simulink model "Model_Maxime"  (R2023b)
settings: Solver=VariableStepAuto  StartTime=0.0  StopTime=T_tot  FixedStep=1e-6  MaxStep=1/50/100  RelTol=1e-3
values from neighbouring files (symbols this model uses):
  B = 0.0129    [PARAMETERS_MODEL_GR2.m]    (also in Parameters.m; Parameters_Chloe.m)
  d_duration_down_slope = 1    [Parameters.m]    (also in Parameters_Chloe.m)
  d_duration_upslope = 1    [Parameters.m]    (also in Parameters_Chloe.m)
  d_start = 0.5    [Parameters.m]    (also in Parameters_Chloe.m)
  d_start_down_slope = 8    [Parameters.m]    (also in Parameters_Chloe.m)
  d_start_down_step = 11    [Parameters.m]    (also in Parameters_Chloe.m)
  d_start_upslope = 1    [Parameters.m]    (also in Parameters_Chloe.m)
  d_start_upstep = 4    [Parameters.m]    (also in Parameters_Chloe.m)
  d_stop = 2    [Parameters.m]    (also in Parameters_Chloe.m)
  f_r = 50    [PARAMETERS_MODEL_GR2.m]    (also in Parameters.m; Parameters_Chloe.m)
  J = 0.2799    [PARAMETERS_MODEL_GR2.m]    (also in Parameters.m; Parameters_Chloe.m)
  Ki = Ki*Ts_w    (= 0.00645)    [PARAMETERS_MODEL_GR2.m]    (also in Parameters.m = 0.37903125; Parameters_Chloe.m = 1.04185)
  Kp = Kp + Ki*Ts_w/2    (= 210.627975)    [PARAMETERS_MODEL_GR2.m]    (also in Parameters.m = 2.463703125; Parameters_Chloe.m = 6.772025)
  L_lr = 1.8e-3    (= 0.0018)    [PARAMETERS_MODEL_GR2.m]    (also in Parameters.m; Parameters_Chloe.m)
  L_ls = 1.8e-3    (= 0.0018)    [PARAMETERS_MODEL_GR2.m]    (also in Parameters.m; Parameters_Chloe.m)
  N_steady = N_r    (= 1460)    [PARAMETERS_MODEL_GR2.m]    (also in Parameters.m = 1450; Parameters_Chloe.m = 1450)
  P = 4    [PARAMETERS_MODEL_GR2.m]    (also in Parameters.m; Parameters_Chloe.m)
  P_r = 19e3    (= 19000)    [PARAMETERS_MODEL_GR2.m]    (also in Parameters.m; Parameters_Chloe.m)
  Phi_n = V_s/w_s    [PARAMETERS_MODEL_GR2.m]    (also in Parameters.m = V_r*sqrt(2)/sqrt(3)/(2*pi*f_r); Parameters_Chloe.m = V_r*sqrt(2)/sqrt(3)/(2*pi*f_r))
  R_r = 0.1091    [PARAMETERS_MODEL_GR2.m]    (also in Parameters.m; Parameters_Chloe.m)
  R_s = 0.0629    [PARAMETERS_MODEL_GR2.m]    (also in Parameters.m; Parameters_Chloe.m)
  T_sat = 0.9*T_max    [PARAMETERS_MODEL_GR2.m]    (also in Parameters.m = 124.271667894; Parameters_Chloe.m = 621.358339468)
  T_tot = 8    [PARAMETERS_MODEL_GR2.m]    (also in Parameters.m = 13; Parameters_Chloe.m = 13)
  Ts = 5e-6    (= 5e-06)    [PARAMETERS_MODEL_GR2.m]    (also in Parameters.m = 1e-05; Parameters_Chloe.m = 1e-05)
  Ts_w = 1/fs_w    (= 0.000664451827243)    [PARAMETERS_MODEL_GR2.m]    (also in Parameters.m = 0.0410256410256; Parameters_Chloe.m = 0.0149253731343)
  U_ac = 380    [PARAMETERS_MODEL_GR2.m]    (also in Parameters.m; Parameters_Chloe.m)
  V_f_in = [-f_r-1 -f_r -f_min 0 f_min f_r f_r+1]*2*pi    [PARAMETERS_MODEL_GR2.m]    (also in Parameters.m; Parameters_Chloe.m)
  V_f_out = [V_s V_s V_min V_min V_min V_s V_s]/V_s    [PARAMETERS_MODEL_GR2.m]    (also in Parameters.m = [V_r V_r V_min V_min V_min V_r V_r]/V_r; Parameters_Chloe.m = [V_r V_r V_min V_min V_min V_r V_r]/V_r)
  V_r = 400    [PARAMETERS_MODEL_GR2.m]    (also in Parameters.m; Parameters_Chloe.m)
undefined symbols (not defined in the file or in its folder): d_steady_start, d_steady_stop
libraries: spsDiodeLib x6, spsIGBTLib x6, simulink x4, spsAsynchronousMachineSIUnitsLib x1, spsDCVoltageSourceLib x1, slpidlib x1, spsMosfetLib x1, spsThreePhaseVIMeasurementLib x1, spsTriangleGeneratorLib x1, sps_lib x1
settings Model: Creator=dimit  LastModifiedBy=dimit

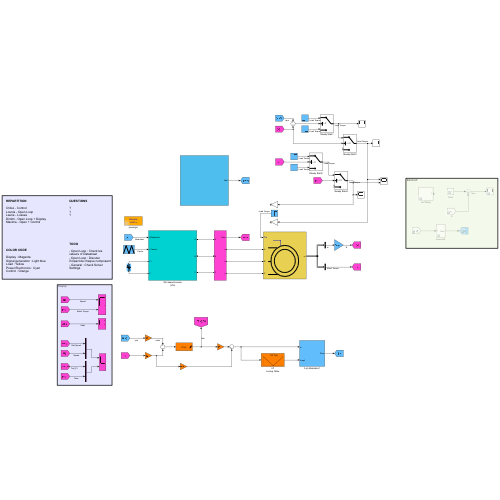
[thumbnail: Simulink's stored preview of the top-level diagram]
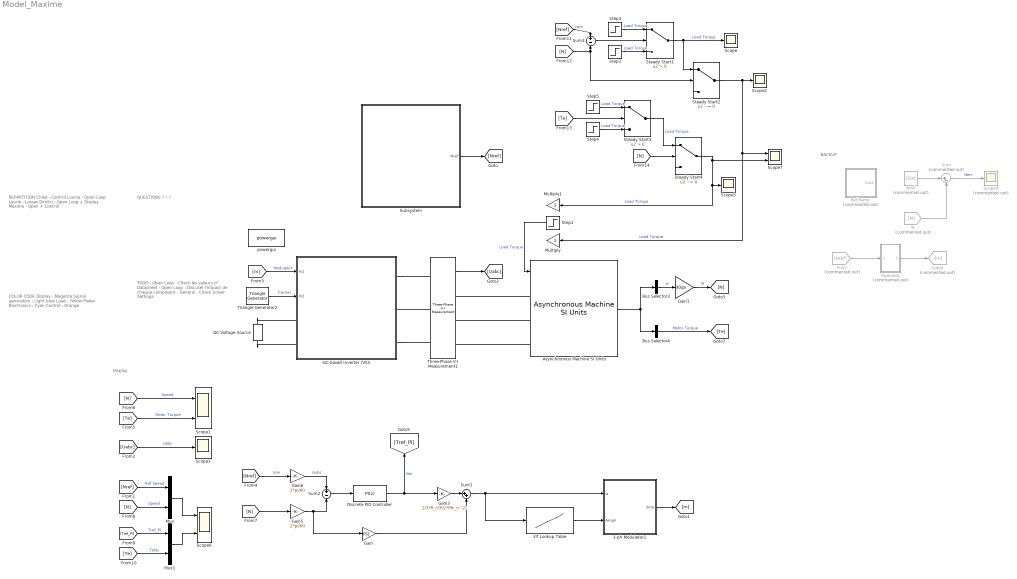
== system Model_Maxime ==
  note: BACKUP
  note: Display
  note: COLOR CODE
      |
      | Display : Magenta
      | Signal generation : Light blue
      | Load : Yellow
      | Power Electronics : Cyan
      | Control : Orange
  note: QUESTIONS
      |
      | ?
      | ?
      | ?
  note: TODO
      |
      | - Open Loop : Check les valeurs cf Datasheet
      | - Open Loop : Discuter l'impact de chaque composant
      | - General : Check Solver Settings
  note: REPARTITION
      |
      | Chloé - Control
      | Lounia - Open Loop
      | Laurie - Losses
      | Dimitri - Open Loop + Display
      | Maxime - Open + Control
  3-ph Modulator1 : Subsystem
  Asynchronous Machine SI Units : spsAsynchronousMachineSIUnitsLib/Asynchronous Machine SI Units  RotorType=Squirrel-cage  PresetModel=No  MechanicalLoad=Torque Tm  ShowDetailedParameters=on  ReferenceFrame=Rotor  Units=SI  MeasurementBus=off  NominalParameters=[P_r V_r f_r]  VoltageRatio=1  Stator=[R_s L_ls]  Rotor=[R_r L_lr]  Cage1=[0.4155 0.002066]  Cage2=[0.4168 0.0003495]  Lm=L_m  Mechanical=[J B P/2]  PolePairs=2  InitialConditions=[1 0 0 0 0 0 0 0]  SimulateSaturation=off  Saturation=[14.03593122, 27.81365428, 53.79336849, 72.68890987, 97.98006896, 148.6815601, 215.7428561, 302.9841135, 428.7778367 ; 230, 322, 414, 460, 506, 552, 598, 644, 690]  LoadFlowParameters=1492000  TsPowergui=0  TsBlock=-1  IterativeModel=Trapezoidal non iterative  IterativeDiscreteModel=Trapezoidal non iterative  Pmec=1.492e+006
  Bus Selector3 : BusSelector  OutputSignals=Mechanical.Rotor speed (wm)  OutputAsBus=on
  Bus Selector4 : BusSelector  OutputSignals=Mechanical.Electromagnetic torque Te (N*m)  OutputAsBus=on
  DC Voltage Source : spsDCVoltageSourceLib/DC Voltage Source  Amplitude=3*sqrt(2)/pi * U_ac  Measurements=None
  Discrete PID Controller : slpidlib/PID Controller  Controller=PI  Form=Parallel  TimeDomain=Discrete-time  UseExternalTs=off  SampleTime=Ts_w  IntegratorMethod=Forward Euler  FilterMethod=Forward Euler  ControllerParametersSource=internal  P=Kp  I=Ki  UseKiTs=off  D=0  N=100  UseFilter=on  TunerSelectOption=Transfer Function Based (PID Tuner App)  InitialConditionSource=internal  InitialConditionForIntegrator=0  InitialConditionForFilter=0  DifferentiatorICPrevScaledInput=0  ExternalReset=none  TrackingMode=off  Kt=1  LimitOutput=on  SatLimitsSource=internal  UpperSaturationLimit=T_sat  LowerSaturationLimit=-T_sat  LinearizeAsGain=off  AntiWindupMode=back-calculation  Kb=1/Kp  LimitIntegrator=off  UpperIntegratorSaturationLimit=inf  LowerIntegratorSaturationLimit=-inf  POutMin=[]  POutMax=[]  IOutMin=[]  IOutMax=[]  DOutMin=[]  DOutMax=[]  NOutMin=[]  NOutMax=[]  SumOutMin=[]  SumOutMax=[]  SaturationOutMin=[]  SaturationOutMax=[]  PParamMin=[]  PParamMax=[]  IParamMin=[]  IParamMax=[]  DParamMin=[]  DParamMax=[]  NParamMin=[]  NParamMax=[]  KbParamMin=[]  KbParamMax=[]  KtParamMin=[]  KtParamMax=[]  KbOutMin=[]  KbOutMax=[]  KtOutMin=[]  KtOutMax=[]  IntegratorOutMin=[]  IntegratorOutMax=[]  FilterOutMin=[]  FilterOutMax=[]  SumI1OutMin=[]  SumI1OutMax=[]  SumI2OutMin=[]  SumI2OutMax=[]  SumI3OutMin=[]  SumI3OutMax=[]  SumI4OutMin=[]  SumI4OutMax=[]  SumDOutMin=[]  SumDOutMax=[]  DifferentiatorOutMin=[]  DifferentiatorOutMax=[]  FilterDiffOutCoefMin=[]  FilterDiffOutCoefMax=[]  ReciprocalOutMin=[]  ReciprocalOutMax=[]  SumDenOutMin=[]  SumDenOutMax=[]  SumNumOutMin=[]  SumNumOutMax=[]  DivideOutMin=[]  DivideOutMax=[]  UdiffTsProdOutMin=[]  UdiffTsProdOutMax=[]  NTsProdOutMin=[]  NTsProdOutMax=[]  UintegralTsProdOutMin=[]  UintegralTsProdOutMax=[]  UngainTsProdOutMin=[]  UngainTsProdOutMax=[]  ClampingZeroOutDataTypeStr=Inherit: Inherit via back propagation  ClampingZeroOutMin=[]  ClampingZeroOutMax=[]  FilterDenConstantOutDataTypeStr=Inherit: Inherit via back propagation  FilterDenConstantOutMin=[]  FilterDenConstantOutMax=[]  PCopyOutDataTypeStr=Inherit: Inherit via back propagation  PCopyOutMin=[]  PCopyOutMax=[]  NCopyOutDataTypeStr=Inherit: Inherit via back propagation  NCopyOutMin=[]  NCopyOutMax=[]  IntegratorContinuousStateAttributes=''  IntegratorStateMustResolveToSignalObject=off  IntegratorRTWStateStorageClass=Auto  FilterContinuousStateAttributes=''  FilterStateMustResolveToSignalObject=off  FilterRTWStateStorageClass=Auto  ParallelPVariant=InternalParameters  IdealPVariant=Disabled  IVariant=InternalParameters  DVariant=Disabled  IntegratorVariant=Discrete  SatVariant=Enabled  AWVariant=BackCalculation  PCopyVariant=Disabled  TRVariant=Disabled  FdbkBlocksVariant=Forward  IdealPFdbkVariant=Disabled  SatFdbkVariant=Disabled  DerivativeFilterVariant=Disabled  NVariant=Disabled  NCopyVariant=Disabled_SignalSpec  FilterICVariant=Disabled  IntegratorICVariant=InternalICs  ExternalResetVariant=Disabled  TRSumVariant=Passthrough  SumFdbkVariant=Disabled  SumVariant=Sum_PI  TsampFilterVariant=InternalTs  TsampNgainVariant=Passthrough  TsampIntegralVariant=Disabled_SignalSpec  ExternalSaturationOutDataTypeStr=Inherit: Same as second input
      settings: LibrarySourceBlock=simulink/Discrete/Discrete PID Controller
  From : From  Commented=on  GotoTag=Nref
  Gain : Gain  Gain=P/2
  Gain1 : Gain  Gain=30/pi
  Gain3 : Gain  Gain=2/3*R_r/(P/2*Phi_n^2)
  Gain5 : Gain  Gain=2*pi/60
  Gain6 : Gain  Gain=2*pi/60
  Goto4 : Goto  Commented=on  GotoTag=m
  Multiply : Gain
  Multiply1 : Gain
  Mux : Mux  Inputs=2
  Mux1 : Mux  Inputs=2
  N : From  Commented=on  GotoTag=N
  Nref : Constant  Commented=on  Value=1500
  Openloop : Subsystem  Commented=on
  Ref Ramp : Subsystem  Commented=on
  Scope{,2..3,5} (4 alike) : Scope
  Scope1 : Scope  NumInputPorts=2
  Scope4 : Scope  Commented=on
  Scope6 : Scope  NumInputPorts=2
  Scope7 : Scope  NumInputPorts=2
  SiC-based Inverter (VSI) : Subsystem
  Steady Start1 : Switch  Criteria=u2 > Threshold  SaturateOnIntegerOverflow=off  InputSameDT=off
  Steady Start2 : Switch  Criteria=u2 ~= 0  SaturateOnIntegerOverflow=off  InputSameDT=off
  Steady Start3 : Switch  Criteria=u2 > Threshold  SaturateOnIntegerOverflow=off  InputSameDT=off
  Steady Start4 : Switch  Criteria=u2 ~= 0  SaturateOnIntegerOverflow=off  InputSameDT=off
  Step1 : Step  After=10  SampleTime=0
  Step2 : Step  After=-10  SampleTime=0
  Step3 : Step  After=10  SampleTime=0
  Step4 : Step  After=-10  SampleTime=0
  Step5 : Step  After=10  SampleTime=0
  Subsystem : Subsystem
  Sum : Sum  Commented=on  Inputs=|+-
  Sum1 : Sum  Inputs=|++
  Sum2 : Sum  Inputs=+|-
  Sum3 : Sum  Inputs=+|-
  Three-Phase V-I Measurement1 : spsThreePhaseVIMeasurementLib/Three-Phase V-I Measurement  VoltageMeasurement=phase-to-phase  SetLabelV=off  LabelV=Vabc  Vpu=off  VpuLL=off  CurrentMeasurement=no  SetLabelI=off  LabelI=Iabc  Ipu=off  Pbase=100e6  Vbase=500e3  OutputType=Complex  PhasorSimulation=off  PSBequivalent=0
  Triangle Generator2 : spsTriangleGeneratorLib/Triangle Generator  Freq=f_switch  Phase=0  Ts=0
  V/f Lookup Table : Lookup_n-D  NumberOfTableDimensions=1  BreakpointsForDimension1=V_f_in  Table=V_f_out  InternalRulePriority=Speed  RndMeth=Simplest
  powergui : sps_lib/powergui  Priority=1  SimulationMode=Discrete  SampleTime=Ts  frequency=60  Iterations=50  frequencyindice=0  Pbase=100e6  ErrMax=1e-4  UnitsV=kV  UnitsW=MW  buscounter=0  FunctionMessages=off  echomessages=off  EnableUseOfTLC=off  CurrentSourceSwitches=off  DisableSnubberDevices=off  DisableRonSwitches=off  DisableVfSwitches=off  DisplayEquations=off  AutomaticDiscreteSolvers=off  SolverType=Tustin/Backward Euler (TBE)  Interpol=off  ExternalGateDelay=off  methode=off  Ts=100  x0status=blocks  SPID=on  SwTol=0  HookPort=off  NonlinearTolerance=1e-4  nMaxIteration=100  ContinueOnMaxIteration=off  RestoreLinks=warning  ResistiveCurrentMeasurement=off  Frange=[0:2:500]  Ylog=off  Xlog=on  ShowGrid=off  save=off  variable=ZData  structure=0  ZoomFFT=off  StartTime=0.0  cycles=1  DisplayStyle=1  fundamental=60  FreqAxis=off  MaxFrequency=1000  frequencyindicesteady=1  RmsSteady=1  display=off
  wires:
  Triangle Generator2/1 -> SiC-based Inverter (VSI)/2(In2)  "Carrier"
  [m] -> SiC-based Inverter (VSI)/1(In1)  "Modulator"
  Three-Phase V-I Measurement1/1 -> [Uabc]
  Asynchronous Machine SI Units/1 -> Bus Selector4/1, Bus Selector3/1
  Bus Selector4/1 -> [Te]  "Motor Torque"
  Bus Selector3/1 -> Gain1/1  "w"
  Gain1/1 -> [N]  "N"
  [Te] -> Scope1/2  "Motor Torque"
  [N] -> Scope1/1  "Speed"
  [Uabc] -> Scope3/1  "Uabc"
  Nref/1 -> Sum/1
  N/1 -> Sum/2
  Sum/1 -> Scope4/1  "Nerr"
  V/f Lookup Table/1 -> 3-ph Modulator1/2(Ampli)
  3-ph Modulator1/1(Sine) -> [m]
  From/1 -> Openloop/1(In1)
  Openloop/1(Sine) -> Goto4/1
  [N] -> Gain5/1
  Gain5/1 -> Gain/1, Sum2/2
  Gain/1 -> Sum1/2
  [Nref] -> Gain6/1  "rpm"
  Gain3/1 -> Sum1/1
  Sum2/1 -> Discrete PID Controller/1
  Discrete PID Controller/1 -> Gain3/1, [Tref_PI]  "Nm"
  Gain6/1 -> Sum2/1  "rad/s"
  Sum1/1 -> V/f Lookup Table/1, 3-ph Modulator1/1(w)
  [Nref] -> Mux/1  "Ref Speed"
  [N] -> Mux/2  "Speed"
  Mux/1 -> Scope6/1
  [Tref_PI] -> Mux1/1  "Tref_PI"
  [Te] -> Mux1/2  "Telec"
  Mux1/1 -> Scope6/2
  Subsystem/1(Nref) -> [Nref]
  [Nref] -> Sum3/1  "rpm"
  [N] -> Steady Start2/2, Sum3/2
  Sum3/1 -> Steady Start1/2
  Step2/1 -> Steady Start1/3  "Load Torque"
  Step3/1 -> Steady Start1/1  "Load Torque"
  Steady Start1/1 -> Steady Start2/1, Scope/1  "Load Torque"
  Steady Start2/1 -> Multiply/1, Scope7/1, Scope2/1  "Load Torque"
  Step4/1 -> Steady Start3/3  "Load Torque"
  [Te] -> Steady Start3/2
  Step5/1 -> Steady Start3/1  "Load Torque"
  [N] -> Steady Start4/2
  Steady Start3/1 -> Steady Start4/1  "Load Torque"
  Steady Start4/1 -> Scope5/1, Multiply1/1, Scope7/2  "Load Torque"
  Step1/1 -> Asynchronous Machine SI Units/1  "Load Torque"
  connections:
  Three-Phase V-I Measurement1/LConn2 -- SiC-based Inverter (VSI)/RConn2
  SiC-based Inverter (VSI)/RConn3 -- Three-Phase V-I Measurement1/LConn3
  Asynchronous Machine SI Units/LConn1 -- Three-Phase V-I Measurement1/RConn1
  Asynchronous Machine SI Units/LConn2 -- Three-Phase V-I Measurement1/RConn2
  Asynchronous Machine SI Units/LConn3 -- Three-Phase V-I Measurement1/RConn3
  DC Voltage Source/RConn1 -- SiC-based Inverter (VSI)/LConn1
  DC Voltage Source/LConn1 -- SiC-based Inverter (VSI)/LConn2
  SiC-based Inverter (VSI)/RConn1 -- Three-Phase V-I Measurement1/LConn1

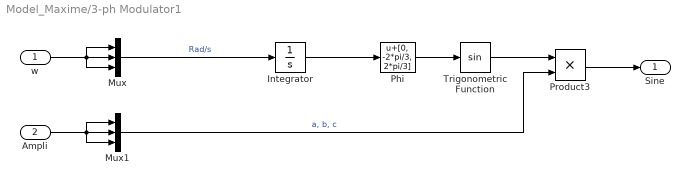
== system Model_Maxime/3-ph Modulator1 ==
  w : Inport
  Ampli : Inport  Port=2
  Integrator : Integrator
  Mux : Mux  Inputs=3
  Mux1 : Mux  Inputs=3
  Phi : Bias  Bias=[0, -2*pi/3, 2*pi/3]  SaturateOnIntegerOverflow=off
  Product3 : Product
  Trigonometric Function : Trigonometry
  Sine : Outport
  wires:
  Integrator/1 -> Phi/1
  Trigonometric Function/1 -> Product3/1
  Mux/1 -> Integrator/1  "Rad/s"
  Mux1/1 -> Product3/2  "a, b, c"
  Ampli/1 -> Mux1/1, Mux1/3, Mux1/2
  w/1 -> Mux/3, Mux/2, Mux/1
  Phi/1 -> Trigonometric Function/1
  Product3/1 -> Sine/1

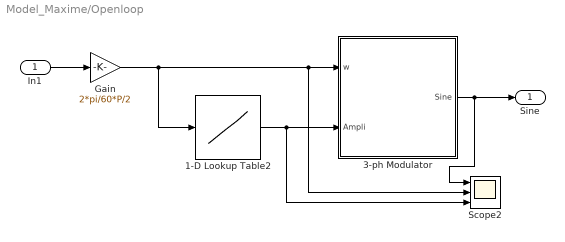
== system Model_Maxime/Openloop ==
  In1 : Inport
  1-D Lookup Table2 : Lookup_n-D  NumberOfTableDimensions=1  BreakpointsForDimension1=V_f_in  Table=V_f_out  InternalRulePriority=Speed  RndMeth=Simplest
  3-ph Modulator : Subsystem
  Gain : Gain  Gain=2*pi/60*P/2
  Scope2 : Scope  NumInputPorts=3
  Sine : Outport
  wires:
  Gain/1 -> Scope2/2, 3-ph Modulator/1(w), 1-D Lookup Table2/1
  3-ph Modulator/1(Sine) -> Sine/1, Scope2/1
  1-D Lookup Table2/1 -> Scope2/3, 3-ph Modulator/2(Ampli)
  In1/1 -> Gain/1

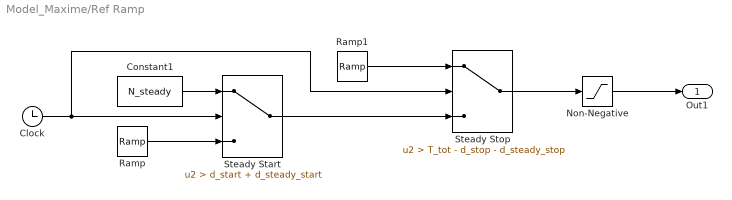
== system Model_Maxime/Ref Ramp ==
  Clock : Clock
  Constant1 : Constant  Value=N_steady
  Non-Negative : Saturate  UpperLimit=inf  LowerLimit=0
  Ramp : simulink/Sources/Ramp  slope=N_steady/d_steady_start  start=d_start  InitialOutput=0
  Ramp1 : simulink/Sources/Ramp  slope=-N_steady/d_steady_stop  start=T_tot - d_stop - d_steady_stop  InitialOutput=N_steady
  Steady Start : Switch  Criteria=u2 > Threshold  Threshold=d_start + d_steady_start  SaturateOnIntegerOverflow=off  InputSameDT=off
  Steady Stop : Switch  Criteria=u2 > Threshold  Threshold=T_tot - d_stop - d_steady_stop  SaturateOnIntegerOverflow=off  InputSameDT=off
  Out1 : Outport
  wires:
  Clock/1 -> Steady Start/2, Steady Stop/2
  Ramp/1 -> Steady Start/3
  Steady Stop/1 -> Non-Negative/1
  Steady Start/1 -> Steady Stop/3
  Ramp1/1 -> Steady Stop/1
  Constant1/1 -> Steady Start/1
  Non-Negative/1 -> Out1/1

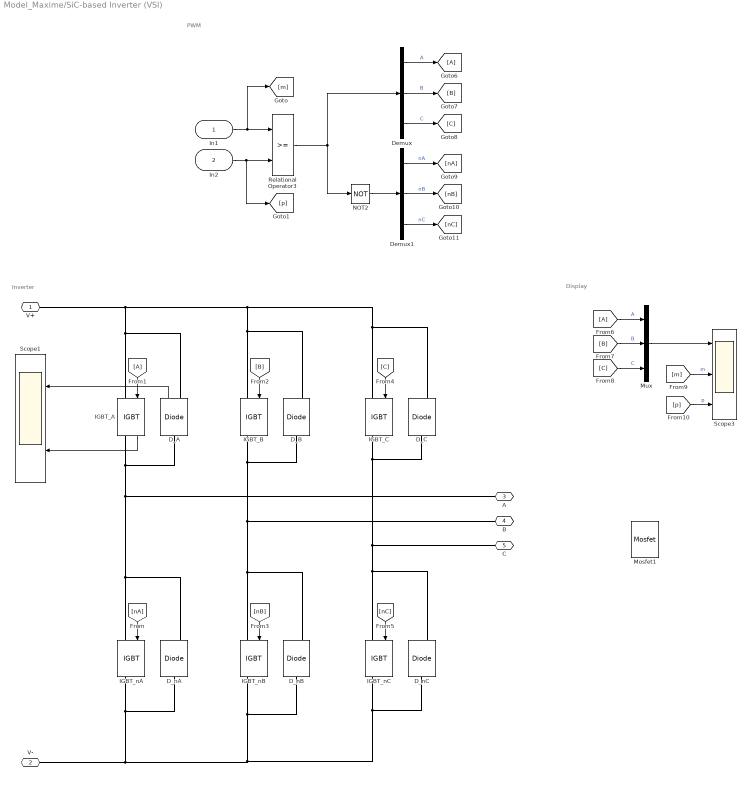
== system Model_Maxime/SiC-based Inverter (VSI) ==
  note: Display
  note: PWM
  note: Inverter
  In1 : Inport
  In2 : Inport  Port=2
  D_A : spsDiodeLib/Diode  Ron=R_d_inv  Lon=L_on_inv  Vf=V_f_inv  IC=0  UseSnubber=0  Rs=R_snub_inv  Cs=C_snub_inv  Measurements=on
  D_B : spsDiodeLib/Diode  Ron=R_d_inv  Lon=L_on_inv  Vf=V_f_inv  IC=0  UseSnubber=0  Rs=R_snub_inv  Cs=C_snub_inv  Measurements=on
  D_C : spsDiodeLib/Diode  Ron=R_d_inv  Lon=L_on_inv  Vf=V_f_inv  IC=0  UseSnubber=0  Rs=R_snub_inv  Cs=C_snub_inv  Measurements=on
  D_nA : spsDiodeLib/Diode  Ron=R_d_inv  Lon=L_on_inv  Vf=V_f_inv  IC=0  UseSnubber=0  Rs=R_snub_inv  Cs=C_snub_inv  Measurements=on
  D_nB : spsDiodeLib/Diode  Ron=R_d_inv  Lon=L_on_inv  Vf=V_f_inv  IC=0  UseSnubber=0  Rs=R_snub_inv  Cs=C_snub_inv  Measurements=on
  D_nC : spsDiodeLib/Diode  Ron=R_d_inv  Lon=L_on_inv  Vf=V_f_inv  IC=0  UseSnubber=0  Rs=R_snub_inv  Cs=C_snub_inv  Measurements=on
  Demux : Demux  Outputs=3
  Demux1 : Demux  Outputs=3
  From1 : From
  From6 : From
  Goto6 : Goto
  IGBT_A : spsIGBTLib/IGBT  Ron=R_on_inv  Lon=L_on_inv  Vf=V_f_inv  Tf=1e-6  Tt=2e-6  IC=0  Rs=R_snub_inv  Cs=C_snub_inv  Measurements=on
  IGBT_B : spsIGBTLib/IGBT  Ron=R_on_inv  Lon=L_on_inv  Vf=V_f_inv  Tf=1e-6  Tt=2e-6  IC=0  Rs=R_snub_inv  Cs=C_snub_inv  Measurements=on
  IGBT_C : spsIGBTLib/IGBT  Ron=R_on_inv  Lon=L_on_inv  Vf=V_f_inv  Tf=1e-6  Tt=2e-6  IC=0  Rs=R_snub_inv  Cs=C_snub_inv  Measurements=on
  IGBT_nA : spsIGBTLib/IGBT  Ron=R_on_inv  Lon=L_on_inv  Vf=V_f_inv  Tf=1e-6  Tt=2e-6  IC=0  Rs=R_snub_inv  Cs=C_snub_inv  Measurements=on
  IGBT_nB : spsIGBTLib/IGBT  Ron=R_on_inv  Lon=L_on_inv  Vf=V_f_inv  Tf=1e-6  Tt=2e-6  IC=0  Rs=R_snub_inv  Cs=C_snub_inv  Measurements=on
  IGBT_nC : spsIGBTLib/IGBT  Ron=R_on_inv  Lon=L_on_inv  Vf=V_f_inv  Tf=1e-6  Tt=2e-6  IC=0  Rs=R_snub_inv  Cs=C_snub_inv  Measurements=on
  Mosfet1 : spsMosfetLib/Mosfet  Ron=R_on_inv  Lon=L_on_inv  Rd=R_d_inv  Vfd=V_f_inv  IC=0  Rs=R_snub_inv  Cs=C_snub_inv  Measurements=on
  Mux : Mux  Inputs=3
  NOT2 : Logic  Operator=NOT  AllPortsSameDT=off  OutDataTypeStr=boolean
  Relational Operator3 : RelationalOperator  OutDataTypeStr=boolean  RndMeth=Simplest  InputSameDT=off
  Scope1 : Scope  NumInputPorts=2
  Scope3 : Scope  NumInputPorts=3
  V+ : PMIOPort  Side=Left
  V- : PMIOPort  Port=2  Side=Left
  A : PMIOPort  Port=3  Side=Right
  B : PMIOPort  Port=4  Side=Right
  C : PMIOPort  Port=5  Side=Right
  wires:
  [nA] -> IGBT_nA/1
  [C] -> IGBT_C/1
  [nB] -> IGBT_nB/1
  From1/1 -> IGBT_A/1
  [nC] -> IGBT_nC/1
  In2/1 -> Relational Operator3/2, [p]
  [B] -> IGBT_B/1
  In1/1 -> [m], Relational Operator3/1
  Relational Operator3/1 -> NOT2/1, Demux/1
  Demux/1 -> Goto6/1  "A"
  Demux/2 -> [B]  "B"
  Demux/3 -> [C]  "C"
  Demux1/3 -> [nC]  "nC"
  Demux1/1 -> [nA]  "nA"
  Demux1/2 -> [nB]  "nB"
  NOT2/1 -> Demux1/1
  From6/1 -> Mux/1  "A"
  [B] -> Mux/2  "B"
  [C] -> Mux/3  "C"
  Mux/1 -> Scope3/1
  [m] -> Scope3/2  "m"
  [p] -> Scope3/3  "p"
  IGBT_A/1 -> Scope1/2
  D_A/1 -> Scope1/1
  connections:
  V+/RConn1 -- D_C/RConn1 -- IGBT_C/LConn1 -- D_B/RConn1 -- IGBT_B/LConn1 -- D_A/RConn1 -- IGBT_A/LConn1
  V-/RConn1 -- D_nB/LConn1 -- IGBT_nB/RConn1 -- D_nC/LConn1 -- IGBT_nC/RConn1 -- IGBT_nA/RConn1 -- D_nA/LConn1
  A/RConn1 -- IGBT_nA/LConn1 -- D_nA/RConn1 -- D_A/LConn1 -- IGBT_A/RConn1
  IGBT_B/RConn1 -- D_B/LConn1 -- D_nB/RConn1 -- IGBT_nB/LConn1 -- B/RConn1
  IGBT_C/RConn1 -- D_C/LConn1 -- D_nC/RConn1 -- IGBT_nC/LConn1 -- C/RConn1

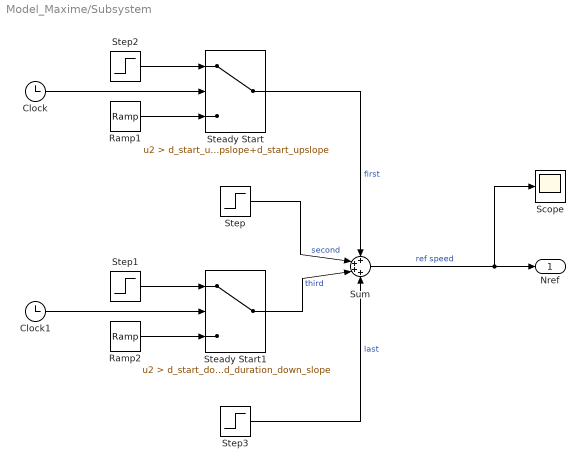
== system Model_Maxime/Subsystem ==
  Clock : Clock
  Clock1 : Clock
  Ramp1 : simulink/Sources/Ramp  slope=750/d_duration_upslope  start=d_start_upslope  InitialOutput=0
  Ramp2 : simulink/Sources/Ramp  slope=-750/d_duration_down_slope  start=d_start_down_slope  InitialOutput=0
  Scope : Scope
  Steady Start : Switch  Criteria=u2 > Threshold  Threshold=d_start_upslope+d_start_upslope  SaturateOnIntegerOverflow=off  InputSameDT=off
  Steady Start1 : Switch  Criteria=u2 > Threshold  Threshold=d_start_down_slope + d_duration_down_slope  SaturateOnIntegerOverflow=off  InputSameDT=off
  Step : Step  Time=d_start_upstep  After=750  SampleTime=0
  Step1 : Step  Time=0  After=-750  SampleTime=0
  Step2 : Step  Time=0  After=750  SampleTime=0
  Step3 : Step  Time=d_start_down_step  After=-750  SampleTime=0
  Sum : Sum  Inputs=++++
  Nref : Outport
  wires:
  Ramp1/1 -> Steady Start/3
  Step2/1 -> Steady Start/1
  Clock/1 -> Steady Start/2
  Steady Start/1 -> Sum/1  "first"
  Step/1 -> Sum/2  "second"
  Sum/1 -> Scope/1, Nref/1  "ref speed"
  Step1/1 -> Steady Start1/1
  Clock1/1 -> Steady Start1/2
  Ramp2/1 -> Steady Start1/3
  Steady Start1/1 -> Sum/3  "third"
  Step3/1 -> Sum/4  "last"

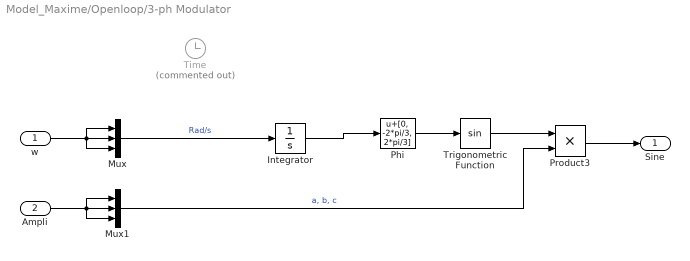
== system Model_Maxime/Openloop/3-ph Modulator ==
  w : Inport
  Ampli : Inport  Port=2
  Integrator : Integrator
  Mux : Mux  Inputs=3
  Mux1 : Mux  Inputs=3
  Phi : Bias  Bias=[0, -2*pi/3, 2*pi/3]  SaturateOnIntegerOverflow=off
  Product3 : Product
  Time : Clock  Commented=on
  Trigonometric Function : Trigonometry
  Sine : Outport
  wires:
  Integrator/1 -> Phi/1
  Trigonometric Function/1 -> Product3/1
  Mux/1 -> Integrator/1  "Rad/s"
  Mux1/1 -> Product3/2  "a, b, c"
  Ampli/1 -> Mux1/1, Mux1/3, Mux1/2
  w/1 -> Mux/3, Mux/2, Mux/1
  Phi/1 -> Trigonometric Function/1
  Product3/1 -> Sine/1
